simulink model "quarter_car_MixedSensitivity"  (R2025b)
settings: Solver=VariableStepAuto  StartTime=0.0  StopTime=30  RelTol=1e-3
values from neighbouring files (symbols this model uses):
  A = [ 0,            1,          0,           -1 ... (first row only)    [Analisi_bode_sistema.m]    (also in H2_LQG_synthesis.m; LQG.m = [ 0,                    1,           0,                    -; LQG_pt2.m = [ 0, 1, 0, -1; LQG_pt2.mat = [0 -57.1428571429 0 400 1 -4.28571428571 0 30 0 0 0 -3600 ..)
  B = [ 0,       0,      0 ... (first row only)    [LQG.m]    (also in LQG_pt2.m = [ 0, 0, 0; LQG_pt2.mat = [0  0  0; 0.00285714285714  0  0; 0  0  -1; -0.02  0.02  3]; Lin_model.m; MIX.m)
  C = [ -ks0/m_s, -bs/m_s,  0,       bs/m_s ... (first row only)    [LQG.m]    (also in LQG_pt2.m = [ -ks0/m_s, -bs/m_s, 0, bs/m_s; LQG_pt2.mat = [-57.1428571429 1 0 400 -4.28571428571 0 0 30 0 0 1 -3600 ..; Lin_model.m; MIX.m = [ -k_s/m_s, -b_s/m_s, 0, b_s/m_s)
  D = [ 1/m_s,   0,      0 ... (first row only)    [LQG.m]    (also in LQG_pt2.m = [ 1/m_s, 0, 0; LQG_pt2.mat = [0.00285714285714  0  0; 0  0  0; 0  0  0; -0.02  0.02  3]; Lin_model.m; MIX.m)
  omega_n1 = 80    [A_quarter_car_parameters.m]    (also in A_uncertain_Plant.m = parameters.omega_n1; Incert_plant.m; LQG.m; LQG_pt2.m)
  tau_1 = 0.005    [A_quarter_car_parameters.m]    (also in LQG.m; LQG_pt2.m; LQG_pt2.mat; Lin_model.m)
  tau_2 = 0.010    (= 0.01)    [A_quarter_car_parameters.m]    (also in LQG.m; LQG_pt2.m; LQG_pt2.mat; Lin_model.m)
  tau_a = 0.025    [A_quarter_car_parameters.m]    (also in A_uncertain_Plant.m = parameters.tau_a; Incert_plant.m; LQG.m; LQG_pt2.m)
  x0_delta_s = 0    [A_quarter_car_parameters.m]    (also in quarter_car_parameters.m)
  x0_delta_t = 0    [A_quarter_car_parameters.m]    (also in quarter_car_parameters.m)
  x0_zs_dot = 0    [A_quarter_car_parameters.m]    (also in quarter_car_parameters.m)
  x0_zu_dot = 0    [A_quarter_car_parameters.m]    (also in quarter_car_parameters.m)
  zeta_1 = 0.7    [A_quarter_car_parameters.m]    (also in A_uncertain_Plant.m = parameters.zeta_1; Incert_plant.m; LQG.m; LQG_pt2.m)
libraries: cstblocks x4, simulink x1
settings Model: Creator=ettor  LastModifiedBy=ettor

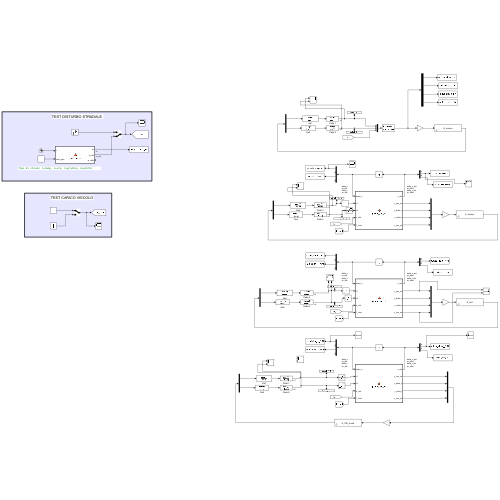
[thumbnail: Simulink's stored preview of the top-level diagram]
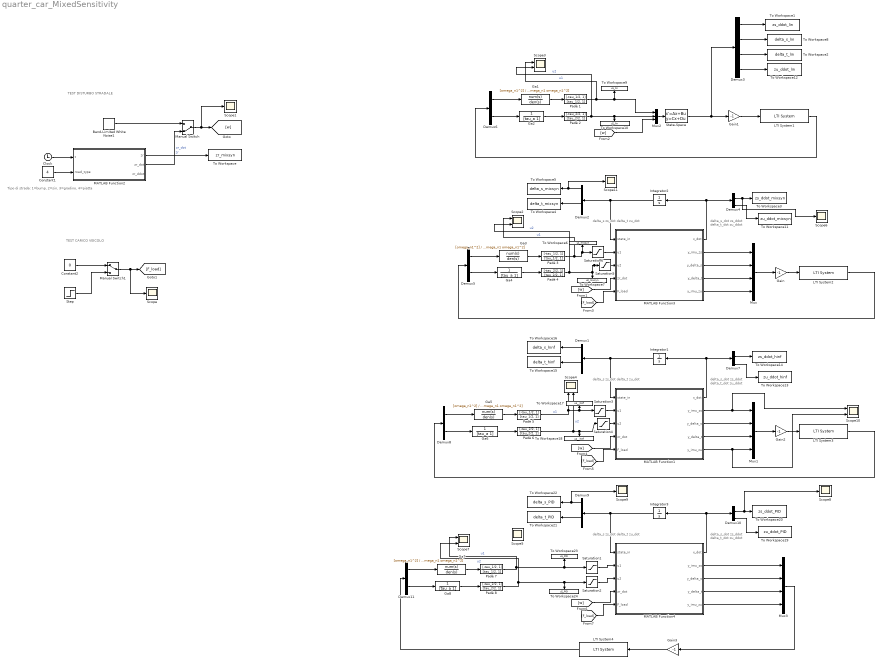
== system quarter_car_MixedSensitivity ==
  note: Tipo di strada: 1=bump, 2=sin, 3=gradino, 4=piatta
  note: delta_s
      | zs_dot
      | delta_t
      | zu_dot
  note: delta_s_dot
      | zs_ddot
      | delta_t_dot
      | zu_ddot
  note: TEST DISTURBO STRADALE
  note: TEST CARICO VEICOLO
  note: delta_s_dot
      | zs_ddot
      | delta_t_dot
      | zu_ddot
  note: delta_s
      | zs_dot
      | delta_t
      | zu_dot
  note: delta_s
      | zs_dot
      | delta_t
      | zu_dot
  note: delta_s_dot
      | zs_ddot
      | delta_t_dot
      | zu_ddot
  Band-Limited White Noise1 : simulink/Sources/Band-Limited White Noise  Cov=[0.0001]  Ts=0.01  seed=[23341]
  Clock : Clock
  Constant1 : Constant  Value=4
  Constant2 : Constant  Value=0
  Demux{1..4,7,9..10} (7 alike) : Demux
  Demux{5..6,8,11} (4 alike) : Demux  Outputs=2
  Ga{1,3,5,7} (4 alike) : TransferFcn  Numerator=[omega_n1^2]  Denominator=[1 2*zeta_1*omega_n1 omega_n1^2]
  Ga{2,4,6,8} (4 alike) : TransferFcn  Denominator=[tau_a 1]
  Gain{,1..3} (4 alike) : Gain  Gain=-1
  Integrator1 : Integrator  InitialCondition=[x0_delta_s; x0_zs_dot; x0_delta_t; x0_zu_dot]
  Integrator2 : Integrator  InitialCondition=[x0_delta_s; x0_zs_dot; x0_delta_t; x0_zu_dot]
  Integrator3 : Integrator  InitialCondition=[x0_delta_s; x0_zs_dot; x0_delta_t; x0_zu_dot]
  LTI System1 : cstblocks/LTI System  sys=K_mixsyn  IC=[]  PadeOrder=0
  LTI System2 : cstblocks/LTI System  sys=K_mixsyn  IC=[]  PadeOrder=0
  LTI System3 : cstblocks/LTI System  sys=K_hinf  IC=[]  PadeOrder=0
  LTI System4 : cstblocks/LTI System  sys=K_PID_tuned  IC=[]  PadeOrder=0
  MATLAB Function1 : MATLAB Function  TreatAsAtomicUnit=on
  MATLAB Function2 : MATLAB Function  TreatAsAtomicUnit=on
  MATLAB Function3 : MATLAB Function  TreatAsAtomicUnit=on
  MATLAB Function4 : MATLAB Function  TreatAsAtomicUnit=on
  Manual Switch : ManualSwitch  CurrentSetting=0
  Manual Switch1 : ManualSwitch
  Mux : Mux
  Mux1 : Mux
  Mux2 : Mux  Inputs=3
  Mux3 : Mux
  Padè {1,3,5,7} (4 alike) : TransferFcn  Numerator=[-tau_1/2, 1]  Denominator=[tau_1/2, 1]
  Padè {2,4,6,8} (4 alike) : TransferFcn  Numerator=[-tau_2/2, 1]  Denominator=[tau_2/2, 1]
  Saturation{1..6} (6 alike) : Saturate  UpperLimit=+3000  LowerLimit=-3000
  Scope{,1,6,8..9,11} (6 alike) : Scope
      Scope settings: ActiveDisplayYMinimum=-1  ActiveDisplayYMaximum=1
      Scope11 settings: ActiveDisplayYMinimum=-1  ActiveDisplayYMaximum=1  DataLoggingVariableName=ScopeData11
      Scope6 settings: ActiveDisplayYMinimum=-1  ActiveDisplayYMaximum=1  DataLoggingVariableName=ScopeData6
      Scope8 settings: DataLoggingVariableName=ScopeData8
      Scope9 settings: ActiveDisplayYMinimum=-1393.9040295799759  ActiveDisplayYMaximum=1770.9119902493803  DataLoggingVariableName=ScopeData9
  Scope{2..5,7,10} (6 alike) : Scope  NumInputPorts=2
      Scope10 settings: ActiveDisplayYMinimum=-1  ActiveDisplayYMaximum=1  DataLoggingVariableName=ScopeData10
      Scope2 settings: ActiveDisplayYMinimum=-1  ActiveDisplayYMaximum=1  DataLoggingVariableName=ScopeData2
      Scope3 settings: ActiveDisplayYMinimum=-1363.5882611538702  ActiveDisplayYMaximum=1563.26057225509  DataLoggingVariableName=ScopeData3
      Scope4 settings: ActiveDisplayYMinimum=-1  ActiveDisplayYMaximum=1  DataLoggingVariableName=ScopeData4
      Scope5 settings: ActiveDisplayYMinimum=-9.2768430147748688E+13  ActiveDisplayYMaximum=4.5138261983738508E+13  DataLoggingVariableName=ScopeData5
      Scope7 settings: ActiveDisplayYMinimum=-8.1374824627813632E+6  ActiveDisplayYMaximum=5.3009031652090633E+6  DataLoggingVariableName=ScopeData7
  State-Space : StateSpace  A=A  B=B  C=C  D=D  InitialCondition=0
  Step : Step  Time=2  After=500  SampleTime=0
  To Workspace : ToWorkspace  VariableName=zr_mixsyn  SaveFormat=Timeseries  SampleTime=-1
  To Workspace1 : ToWorkspace  VariableName=zs_ddot_lin  SaveFormat=Timeseries  SampleTime=-1
  To Workspace10 : ToWorkspace  VariableName=u2_lin  SaveFormat=Timeseries  SampleTime=-1
  To Workspace11 : ToWorkspace  VariableName=zu_ddot_mixsyn  SaveFormat=Timeseries  SampleTime=-1
  To Workspace12 : ToWorkspace  VariableName=zu_ddot_lin  SaveFormat=Timeseries  SampleTime=-1
  To Workspace13 : ToWorkspace  VariableName=zu_ddot_hinf  SaveFormat=Timeseries  SampleTime=-1
  To Workspace14 : ToWorkspace  VariableName=zs_ddot_hinf  SaveFormat=Timeseries  SampleTime=-1
  To Workspace15 : ToWorkspace  VariableName=delta_t_hinf  SaveFormat=Timeseries  SampleTime=-1
  To Workspace16 : ToWorkspace  VariableName=delta_s_hinf  SaveFormat=Timeseries  SampleTime=-1
  To Workspace17 : ToWorkspace  VariableName=u1__hinf  SaveFormat=Timeseries  SampleTime=-1
  To Workspace18 : ToWorkspace  VariableName=u2__hinf  SaveFormat=Timeseries  SampleTime=-1
  To Workspace19 : ToWorkspace  VariableName=zu_ddot_PID  SaveFormat=Timeseries  SampleTime=-1
  To Workspace2 : ToWorkspace  VariableName=delta_t_lin  SaveFormat=Timeseries  SampleTime=-1
  To Workspace20 : ToWorkspace  VariableName=zs_ddot_PID  SaveFormat=Timeseries  SampleTime=-1
  To Workspace21 : ToWorkspace  VariableName=delta_t_PID  SaveFormat=Timeseries  SampleTime=-1
  To Workspace22 : ToWorkspace  VariableName=delta_s_PID  SaveFormat=Timeseries  SampleTime=-1
  To Workspace23 : ToWorkspace  VariableName=u1_PID  SaveFormat=Timeseries  SampleTime=-1
  To Workspace24 : ToWorkspace  VariableName=u2_PID  SaveFormat=Timeseries  SampleTime=-1
  To Workspace3 : ToWorkspace  VariableName=zs_ddot_mixsyn  SaveFormat=Timeseries  SampleTime=-1
  To Workspace4 : ToWorkspace  VariableName=delta_t_mixsyn  SaveFormat=Timeseries  SampleTime=-1
  To Workspace5 : ToWorkspace  VariableName=delta_s_mixsyn  SaveFormat=Timeseries  SampleTime=-1
  To Workspace6 : ToWorkspace  VariableName=u1_mixsyn  SaveFormat=Timeseries  SampleTime=-1
  To Workspace7 : ToWorkspace  VariableName=u2_mixsyn  SaveFormat=Timeseries  SampleTime=-1
  To Workspace8 : ToWorkspace  VariableName=delta_s_lin  SaveFormat=Timeseries  SampleTime=-1
  To Workspace9 : ToWorkspace  VariableName=u1_lin  SaveFormat=Timeseries  SampleTime=-1
  wires:
  Band-Limited White Noise1/1 -> Manual Switch/1
  Constant1/1 -> MATLAB Function2/2(road_type)
  LTI System2/1 -> Demux5/1
  Demux2/1 -> Scope11/1, To Workspace5/1
  Manual Switch/1 -> Scope1/1, [w]
  MATLAB Function3/1(x_dot) -> Demux4/1, Integrator2/1
  [F_load] -> MATLAB Function3/5(F_load)
  Ga3/1 -> Padè 3/1
  Demux5/1 -> Ga3/1
  Demux4/2 -> Scope6/1, To Workspace3/1
  Clock/1 -> MATLAB Function2/1(t)
  Padè 3/1 -> Scope2/1, Saturation6/1, To Workspace6/1  "u1"
  Integrator2/1 -> MATLAB Function3/1(state_in), Demux2/1
  MATLAB Function2/2(zr_dot) -> Manual Switch/2  "zr_dot"
  Demux2/3 -> To Workspace4/1
  Padè 4/1 -> MATLAB Function3/3(u2), Saturation5/1, To Workspace7/1, Scope2/2  "u2"
  Ga4/1 -> Padè 4/1
  Demux5/2 -> Ga4/1
  [w] -> MATLAB Function3/4(zr_dot)
  Manual Switch1/1 -> Scope/1, [F_load]
  Constant2/1 -> Manual Switch1/1
  Step/1 -> Manual Switch1/2
  MATLAB Function3/2(y_imu_zs) -> Mux/1
  MATLAB Function3/3(y_delta_s) -> Mux/2
  MATLAB Function3/4(y_delta_t) -> Mux/3
  MATLAB Function3/5(y_imu_zu) -> Mux/4
  Mux/1 -> Gain/1
  Gain/1 -> LTI System2/1
  MATLAB Function2/1(zr) -> To Workspace/1  "zr"
  Gain1/1 -> LTI System1/1
  Demux6/2 -> Ga2/1
  Padè 2/1 -> Mux2/2, To Workspace10/1, Scope3/2  "u2"
  Ga2/1 -> Padè 2/1
  Padè 1/1 -> Scope3/1, Mux2/1, To Workspace9/1  "u1"
  Demux6/1 -> Ga1/1
  Ga1/1 -> Padè 1/1
  LTI System1/1 -> Demux6/1
  [w] -> Mux2/3
  State-Space/1 -> Demux3/1, Gain1/1
  Mux2/1 -> State-Space/1
  Demux3/2 -> To Workspace8/1
  Demux3/1 -> To Workspace1/1
  Demux3/3 -> To Workspace2/1
  Demux4/4 -> To Workspace11/1
  Demux3/4 -> To Workspace12/1
  MATLAB Function1/4(y_delta_t) -> Mux1/3
  MATLAB Function1/2(y_imu_zs) -> Scope10/1, Mux1/1
  MATLAB Function1/5(y_imu_zu) -> Scope10/2, Mux1/4
  MATLAB Function1/3(y_delta_s) -> Mux1/2
  Gain2/1 -> LTI System3/1
  Demux7/4 -> To Workspace13/1
  Demux8/2 -> Ga6/1
  Padè 6/1 -> Saturation4/1, To Workspace18/1, Scope4/2  "u2"
  Ga6/1 -> Padè 6/1
  Demux1/3 -> To Workspace15/1
  Padè 5/1 -> Saturation3/1, To Workspace17/1, Scope4/1  "u1"
  Integrator1/1 -> MATLAB Function1/1(state_in), Demux1/1
  Mux1/1 -> Gain2/1
  MATLAB Function1/1(x_dot) -> Demux7/1, Integrator1/1
  Demux8/1 -> Ga5/1
  Ga5/1 -> Padè 5/1
  Demux7/2 -> To Workspace14/1
  [F_load] -> MATLAB Function1/5(F_load)
  Demux1/1 -> To Workspace16/1
  [w] -> MATLAB Function1/4(zr_dot)
  LTI System3/1 -> Demux8/1
  MATLAB Function4/4(y_delta_t) -> Mux3/3
  Gain3/1 -> LTI System4/1
  MATLAB Function4/3(y_delta_s) -> Mux3/2
  Integrator3/1 -> MATLAB Function4/1(state_in), Demux9/1
  Demux9/3 -> To Workspace21/1
  Padè 7/1 -> Saturation1/1, To Workspace23/1, Scope7/1  "u1"
  Ga8/1 -> Padè 8/1
  Padè 8/1 -> Saturation2/1, To Workspace24/1, Scope7/2  "u2"
  Demux11/2 -> Ga8/1
  Demux10/4 -> To Workspace19/1
  [w] -> MATLAB Function4/4(zr_dot)
  Demux9/1 -> Scope9/1, To Workspace22/1
  Demux10/2 -> Scope8/1, To Workspace20/1
  Demux11/1 -> Ga7/1
  Mux3/1 -> Gain3/1
  MATLAB Function4/1(x_dot) -> Demux10/1, Integrator3/1
  Ga7/1 -> Padè 7/1
  [F_load] -> MATLAB Function4/5(F_load)
  MATLAB Function4/2(y_imu_zs) -> Mux3/1
  MATLAB Function4/5(y_imu_zu) -> Mux3/4
  LTI System4/1 -> Demux11/1
  Saturation3/1 -> MATLAB Function1/2(u1)
  Saturation4/1 -> MATLAB Function1/3(u2)
  Saturation6/1 -> MATLAB Function3/2(u1)
  Saturation2/1 -> MATLAB Function4/3(u2)
  Saturation1/1 -> MATLAB Function4/2(u1)

== matlab function quarter_car_MixedSensitivity/MATLAB Function1 ==
  data: state_in input; x_dot output; u1 input; u2 input; zr_dot input; F_load input; parameters parameter; y_imu_zs output; y_delta_s output; y_delta_t output; y_imu_zu output
function [x_dot, y_imu_zs, y_delta_s, y_delta_t, y_imu_zu] = quarter_car_NL(state_in, u1, u2, zr_dot, F_load ,parameters)

    delta_s = state_in(1);
    zs_dot = state_in(2);
    delta_t = state_in(3);
    zu_dot = state_in(4);
    
    m_s = parameters.m_s;
    m_u = parameters.m_u;
    ks0 = parameters.ks0;
    alpha = parameters.alpha;
    bs = parameters.bs;
    kt = parameters.kt;
    bt = parameters.bt;
    
    delta_s_dot = zs_dot - zu_dot;
    delta_t_dot = zu_dot - zr_dot;
    
    Fs = ks0 * delta_s + alpha * delta_s^3 + bs * delta_s_dot;
    Ft = kt * delta_t + bt * delta_t_dot;
    
    
    zs_ddot = (-Fs + u1-F_load) / m_s;
    zu_ddot = (Fs - Ft - u1 + u2) / m_u;
    
    x_dot = [delta_s_dot; zs_ddot; delta_t_dot; zu_ddot];
    
    y_imu_zs = zs_ddot;  
    y_imu_zu = zu_ddot; 
    y_delta_s = delta_s; 
    y_delta_t = delta_t; 

end

== matlab function quarter_car_MixedSensitivity/MATLAB Function4 ==
  data: state_in input; x_dot output; u1 input; u2 input; zr_dot input; F_load input; parameters parameter; y_imu_zs output; y_delta_s output; y_delta_t output; y_imu_zu output
function [x_dot, y_imu_zs, y_delta_s, y_delta_t, y_imu_zu] = quarter_car_NL(state_in, u1, u2, zr_dot, F_load ,parameters)

    delta_s = state_in(1);
    zs_dot = state_in(2);
    delta_t = state_in(3);
    zu_dot = state_in(4);
    
    m_s = parameters.m_s;
    m_u = parameters.m_u;
    ks0 = parameters.ks0;
    alpha = parameters.alpha;
    bs = parameters.bs;
    kt = parameters.kt;
    bt = parameters.bt;
    
    delta_s_dot = zs_dot - zu_dot;
    delta_t_dot = zu_dot - zr_dot;
    
    Fs = ks0 * delta_s + alpha * delta_s^3 + bs * delta_s_dot;
    Ft = kt * delta_t + bt * delta_t_dot;
    
    
    zs_ddot = (-Fs + u1-F_load) / m_s;
    zu_ddot = (Fs - Ft - u1 + u2) / m_u;
    
    x_dot = [delta_s_dot; zs_ddot; delta_t_dot; zu_ddot];
    
    y_imu_zs = zs_ddot;  
    y_imu_zu = zu_ddot; 
    y_delta_s = delta_s; 
    y_delta_t = delta_t; 

end

== matlab function quarter_car_MixedSensitivity/MATLAB Function2 ==
  data: t input; zr output; zr_dot output; zr_ddot output; params parameter; road_type input
function [zr, zr_dot, zr_ddot] = road_profile(t, params, road_type)
%   road_type = 1 bump | 2 sinusoide | 3 gradino | 4 piatta

    switch road_type
        case 1  % ---- BUMP ----

            A = params.A;   % altezza [m]
            L = params.L;   % lunghezza [m]
            v = params.v;   % velocità veicolo [m/s]
            t0 = params.t0; % istante di inizio ostacolo [s]
            T = L / v;      % durata temporale bump
            
            % Il dosso inizia a t0 e finisce a t0 + T
            if t >= t0 && t <= (t0 + T)
                t_rel = t - t0; % Tempo relativo (parte da 0 quando inizia il dosso)
                phi   = 2*pi*v*t_rel / L;
                zr    = (A/2) * (1 - cos(phi));
                zr_dot   = (A*pi*v/L) * sin(phi);
                zr_ddot  = (A*2*pi^2*v^2/L^2) * cos(phi);
            else
                zr = 0;  zr_dot = 0;  zr_ddot = 0;
            end
            
        case 2  % ---- SINUSOIDE ----
            A = params.A;   % ampiezza [m]
            f = params.f;   % frequenza [Hz]
            t0 = params.t0; % istante di inizio ostacolo [s]
            
            % La strada vibra solo dopo t0
            if t >= t0
                t_rel = t - t0; % Tempo relativo
                w = 2*pi*f;
                zr   =  A * sin(w*t_rel);
                zr_dot  =  A * w * cos(w*t_rel);
                zr_ddot = -A * w^2 * sin(w*t_rel);
            else
                zr = 0;  zr_dot = 0;  zr_ddot = 0;
            end
            
        case 3  % ---- GRADINO SMUSSATO ----
            A  = params.A;    % altezza [m]
            t0 = params.t0;   % istante del gradino [s]
            tau = params.tau; % tempo di salita [s]
            
            arg  = (t - t0) / tau;
            zr   = (A/2) * (1 + tanh(arg));
            zr_dot  = (A/(2*tau)) * (sech(arg))^2;
            zr_ddot = -(A/tau^2) * (sech(arg))^2 * tanh(arg);
            
        case 4  % ---- STRADA PIATTA ----
            zr = 0;  zr_dot = 0;  zr_ddot = 0;
            
        otherwise 
            zr = 0;  zr_dot = 0;  zr_ddot = 0;
    end
end

== matlab function quarter_car_MixedSensitivity/MATLAB Function3 ==
  data: state_in input; x_dot output; u1 input; u2 input; zr_dot input; F_load input; parameters parameter; y_imu_zs output; y_delta_s output; y_delta_t output; y_imu_zu output
function [x_dot, y_imu_zs, y_delta_s, y_delta_t, y_imu_zu] = quarter_car_NL(state_in, u1, u2, zr_dot, F_load ,parameters)

    delta_s = state_in(1);
    zs_dot = state_in(2);
    delta_t = state_in(3);
    zu_dot = state_in(4);
    
    m_s = parameters.m_s;
    m_u = parameters.m_u;
    ks0 = parameters.ks0;
    alpha = parameters.alpha;
    bs = parameters.bs;
    kt = parameters.kt;
    bt = parameters.bt;
    
    delta_s_dot = zs_dot - zu_dot;
    delta_t_dot = zu_dot - zr_dot;
    
    Fs = ks0 * delta_s + alpha * delta_s^3 + bs * delta_s_dot;
    Ft = kt * delta_t + bt * delta_t_dot;
    
    
    zs_ddot = (-Fs + u1-F_load) / m_s;
    zu_ddot = (Fs - Ft - u1 + u2) / m_u;
    
    x_dot = [delta_s_dot; zs_ddot; delta_t_dot; zu_ddot];
    
    y_imu_zs = zs_ddot;  
    y_imu_zu = zu_ddot; 
    y_delta_s = delta_s; 
    y_delta_t = delta_t; 

end
